simulink model "DCE_motor6_V2"  (R2025a)
settings: Solver=ode4  StartTime=0.0  StopTime=1  FixedStep=5e-5  RelTol=1e-3
undefined symbols (not defined in the file or in its folder): powergui
libraries: spsControlledVoltageSourceLib x24, spsControlledCurrentSourceLib x24, spsVoltageMeasurementLib x24, slpidlib x24, spspowerguiLib x2, simulink x1
(part 5 of 5)

== system DCE_motor6_V2/powergui1/EquivalentModel22/Sources ==
  Mux : Mux  Inputs=[1 1]
  u : Outport  VectorParamsAs1DForOutWhenUnconnected=off
  wires:
  Mux/1 -> u/1
  [T52_4806_4456650309996] -> Mux/1
  [T69_6431_8097857549454] -> Mux/2

== system DCE_motor6_V2/powergui1/EquivalentModel22/Yout ==
  v,i : Inport
  Demux : Demux  Outputs=1
  tag scope: T65_6117_7580539398846=global
  wires:
  v,i/1 -> Demux/1
  Demux/1 -> [T65_6117_7580539398846]

== system DCE_motor6_V2/powergui1/EquivalentModel23/Sources ==
  Mux : Mux  Inputs=[1 1]
  u : Outport  VectorParamsAs1DForOutWhenUnconnected=off
  wires:
  Mux/1 -> u/1
  [T52_4807_4456647609302] -> Mux/1
  [T68_6383_8137968106251] -> Mux/2

== system DCE_motor6_V2/powergui1/EquivalentModel23/Yout ==
  v,i : Inport
  Demux : Demux  Outputs=1
  tag scope: T64_6069_7569106032292=global
  wires:
  v,i/1 -> Demux/1
  Demux/1 -> [T64_6069_7569106032292]

== system DCE_motor6_V2/powergui1/EquivalentModel24/Sources ==
  Mux : Mux  Inputs=[1 1]
  u : Outport  VectorParamsAs1DForOutWhenUnconnected=off
  wires:
  Mux/1 -> u/1
  [T52_4808_4456787087070] -> Mux/1
  [T69_6432_8095244640554] -> Mux/2

== system DCE_motor6_V2/powergui1/EquivalentModel24/Yout ==
  v,i : Inport
  Demux : Demux  Outputs=1
  tag scope: T65_6118_7577934536865=global
  wires:
  v,i/1 -> Demux/1
  Demux/1 -> [T65_6118_7577934536865]

== system DCE_motor6_V2/powergui1/EquivalentModel3/Sources ==
  Mux : Mux  Inputs=[1 1]
  u : Outport  VectorParamsAs1DForOutWhenUnconnected=off
  wires:
  Mux/1 -> u/1
  [T52_4802_4466065559397] -> Mux/1
  [T68_6378_8149266987715] -> Mux/2

== system DCE_motor6_V2/powergui1/EquivalentModel3/Yout ==
  v,i : Inport
  Demux : Demux  Outputs=1
  tag scope: T64_6064_7580471701128=global
  wires:
  v,i/1 -> Demux/1
  Demux/1 -> [T64_6064_7580471701128]

== system DCE_motor6_V2/powergui1/EquivalentModel4/Sources ==
  Mux : Mux  Inputs=[1 1]
  u : Outport  VectorParamsAs1DForOutWhenUnconnected=off
  wires:
  Mux/1 -> u/1
  [T52_4803_4466210929170] -> Mux/1
  [T69_6427_8106398489851] -> Mux/2

== system DCE_motor6_V2/powergui1/EquivalentModel4/Yout ==
  v,i : Inport
  Demux : Demux  Outputs=1
  tag scope: T65_6113_7589152605399=global
  wires:
  v,i/1 -> Demux/1
  Demux/1 -> [T65_6113_7589152605399]

== system DCE_motor6_V2/powergui1/EquivalentModel5/Sources ==
  Mux : Mux  Inputs=[1 1]
  u : Outport  VectorParamsAs1DForOutWhenUnconnected=off
  wires:
  Mux/1 -> u/1
  [T52_4801_4464269315094] -> Mux/1
  [T68_6378_8149612899368] -> Mux/2

== system DCE_motor6_V2/powergui1/EquivalentModel5/Yout ==
  v,i : Inport
  Demux : Demux  Outputs=1
  tag scope: T64_6064_7580793483403=global
  wires:
  v,i/1 -> Demux/1
  Demux/1 -> [T64_6064_7580793483403]

== system DCE_motor6_V2/powergui1/EquivalentModel6/Sources ==
  Mux : Mux  Inputs=[1 1]
  u : Outport  VectorParamsAs1DForOutWhenUnconnected=off
  wires:
  Mux/1 -> u/1
  [T52_4802_4464129149544] -> Mux/1
  [T69_6427_8106740814706] -> Mux/2

== system DCE_motor6_V2/powergui1/EquivalentModel6/Yout ==
  v,i : Inport
  Demux : Demux  Outputs=1
  tag scope: T65_6113_7589471488212=global
  wires:
  v,i/1 -> Demux/1
  Demux/1 -> [T65_6113_7589471488212]

== system DCE_motor6_V2/powergui1/EquivalentModel7/Sources ==
  Mux : Mux  Inputs=[1 1]
  u : Outport  VectorParamsAs1DForOutWhenUnconnected=off
  wires:
  Mux/1 -> u/1
  [T52_4803_4464131162455] -> Mux/1
  [T68_6379_8146968359069] -> Mux/2

== system DCE_motor6_V2/powergui1/EquivalentModel7/Yout ==
  v,i : Inport
  Demux : Demux  Outputs=1
  tag scope: T64_6065_7578157286736=global
  wires:
  v,i/1 -> Demux/1
  Demux/1 -> [T64_6065_7578157286736]

== system DCE_motor6_V2/powergui1/EquivalentModel8/Sources ==
  Mux : Mux  Inputs=[1 1]
  u : Outport  VectorParamsAs1DForOutWhenUnconnected=off
  wires:
  Mux/1 -> u/1
  [T52_4804_4464275353827] -> Mux/1
  [T69_6428_8104129430716] -> Mux/2

== system DCE_motor6_V2/powergui1/EquivalentModel8/Yout ==
  v,i : Inport
  Demux : Demux  Outputs=1
  tag scope: T65_6114_7586868346154=global
  wires:
  v,i/1 -> Demux/1
  Demux/1 -> [T65_6114_7586868346154]

== system DCE_motor6_V2/powergui1/EquivalentModel9/Sources ==
  Mux : Mux  Inputs=[1 1]
  u : Outport  VectorParamsAs1DForOutWhenUnconnected=off
  wires:
  Mux/1 -> u/1
  [T52_4802_4462362678416] -> Mux/1
  [T68_6379_8147334089506] -> Mux/2

== system DCE_motor6_V2/powergui1/EquivalentModel9/Yout ==
  v,i : Inport
  Demux : Demux  Outputs=1
  tag scope: T64_6065_7578500152954=global
  wires:
  v,i/1 -> Demux/1
  Demux/1 -> [T64_6065_7578500152954]

== matlab function DCE_motor6_V2/joint6/MATLAB Function3 ==
  settings: updateMethod=DISCRETE
  data: iq input; TL_est output; wm input; theta_m input
function TL_est = fcn_Load_Observer(iq, wm, theta_m)
    % 步进电机实时负载转矩观测器 (基于 SVF 动态提取)
    % 控制周期: 5e-5 s

    persistent Ts p_pairs Psi_f B J Td;
    persistent a b alpha;
    persistent wf_p T_drive_f_p;

    if isempty(Ts)
        Ts = 5e-5;
        p_pairs = 50;
        
        % --- 【在此填入你的已知常量】 ---
        Psi_f = 0.0015;      % 已知磁链 (Wb)
        B = 1e-4;           % 已知粘滞摩擦系数 (N.m.s/rad)
        J = 1e-5;          % 已知转动惯量 (kg.m^2) (瞬态极重要！)
        Td = 0.003;          % 齿槽转矩幅值 (N.m) (填你模型里的实际值)
        
        % --- SVF 滤波器设计 ---
        % 截止频率设为 200Hz，足以滤除噪声，同时保留负载突变的动态响应
        f_c = 20;           
        alpha = 2 * pi * f_c;
        a = exp(-alpha * Ts);
        b = 1 - a;

        % 历史状态初始化
        wf_p = 0;
        T_drive_f_p = 0;
    end

    % 1. 计算总电磁生成转矩 Te
    T_main = p_pairs * Psi_f * iq;
    T_detent = -Td * sin(4 * p_pairs * theta_m);
    Te = T_main + T_detent;

    % 2. 计算纯驱动力矩 (扣除摩擦阻力)
    % T_drive = Te - B*w 
    T_drive = Te - B * wm;

    % 3. SVF 低通滤波 (平滑转速和驱动力矩)
    wf = a * wf_p + b * wm;
    T_drive_f = a * T_drive_f_p + b * T_drive;

    % 4. SVF 魔法：提取无噪声的角加速度 (dw/dt)
    dw_dt_est = alpha * (wm - wf_p);

    % 5. 计算实时负载转矩
    % TL = T_drive_filtered - J * (dw/dt)
    TL_est = T_drive_f - J * dw_dt_est;

    % 更新历史状态
    wf_p = wf;
    T_drive_f_p = T_drive_f;
end

== matlab function DCE_motor6_V2/joint6/MATLAB Function4 ==
  settings: updateMethod=DISCRETE  sampleTime=5e-5
  data: pos_ref_rad input; I_mag output; pos_real_rad input; vel_ref_rads input; vel_real_rads input; kp input; kv input; ki input; kd input
function I_mag = dce_controller(pos_ref_rad, pos_real_rad, vel_ref_rads, vel_real_rads, kp, kv, ki, kd)
    % 1. 单位转换
    rad2step = 51200 / (2 * pi); 
    pos_ref = pos_ref_rad * rad2step;
    pos_real = pos_real_rad * rad2step;
    vel_ref = vel_ref_rads * rad2step;
    
    % 【撤销滤波，恢复直接获取平滑的积分反馈速度】
    vel_real = vel_real_rads * rad2step; 
    
    % 3. 模拟 C++ 里的积分累加器
    persistent outputKi integralRound
    if isempty(outputKi)
        outputKi = 0;
        integralRound = 0;
    end
    
    pError = pos_ref - pos_real;
    pError = max(min(pError, 3200), -3200); 
    
    vError = (vel_ref - vel_real) / 128; 
    vError = max(min(vError, 4000), -4000); 
    
    outputKp = kp * pError;
    outputKd = kd * vError;
    
    integralRound = integralRound + (ki * pError + kv * vError);
    outputKi = outputKi + (integralRound / 128);
    integralRound = 0; 
    
    outputKi = max(min(outputKi, 1024000), -1024000); 
    
    output = (outputKp + outputKi + outputKd) / 1024; 
    output = max(min(output, 1000), -1000); 
    I_mag = output / 1000; 
end

== matlab function DCE_motor6_V2/joint6/Park1 ==
  data: Ia input; Id output; Ib input; Theta_elec input; Iq output
function [Id, Iq] = fcn(Ia, Ib, Theta_elec)
    Id =  Ia * cos(Theta_elec) + Ib * sin(Theta_elec);
    Iq = -Ia * sin(Theta_elec) + Ib * cos(Theta_elec);
end

== matlab function DCE_motor6_V2/joint6/Park2 ==
  data: Ia input; Id output; Ib input; Theta_elec input; Iq output
function [Id, Iq] = fcn(Ia, Ib, Theta_elec)
    Id =  Ia * cos(Theta_elec) + Ib * sin(Theta_elec);
    Iq = -Ia * sin(Theta_elec) + Ib * cos(Theta_elec);
end

== matlab function DCE_motor6_V2/joint6/RevPark1 ==
  data: Vq input; Vd input; Va_raw output; Theta_elec input; Vb_raw output
function [Va_raw, Vb_raw] = fcn(Vq, Vd, Theta_elec)
    Va_raw = Vd * cos(Theta_elec) - Vq * sin(Theta_elec);
    Vb_raw = Vd * sin(Theta_elec) + Vq * cos(Theta_elec);
end

== matlab function DCE_motor6_V2/joint2/MATLAB Function2 ==
  settings: updateMethod=DISCRETE  sampleTime=5e-5
  data: pos_ref_rad input; I_mag output; pos_real_rad input; vel_ref_rads input; vel_real_rads input; kp input; kv input; ki input; kd input
function I_mag = dce_controller(pos_ref_rad, pos_real_rad, vel_ref_rads, vel_real_rads, kp, kv, ki, kd)
    % 1. 单位转换
    rad2step = 51200 / (2 * pi); 
    pos_ref = pos_ref_rad * rad2step;
    pos_real = pos_real_rad * rad2step;
    vel_ref = vel_ref_rads * rad2step;
    
    % 【撤销滤波，恢复直接获取平滑的积分反馈速度】
    vel_real = vel_real_rads * rad2step; 
    
    % 3. 模拟 C++ 里的积分累加器
    persistent outputKi integralRound
    if isempty(outputKi)
        outputKi = 0;
        integralRound = 0;
    end
    
    pError = pos_ref - pos_real;
    pError = max(min(pError, 3200), -3200); 
    
    vError = (vel_ref - vel_real) / 128; 
    vError = max(min(vError, 4000), -4000); 
    
    outputKp = kp * pError;
    outputKd = kd * vError;
    
    integralRound = integralRound + (ki * pError + kv * vError);
    outputKi = outputKi + (integralRound / 128);
    integralRound = 0; 
    
    outputKi = max(min(outputKi, 1024000), -1024000); 
    
    output = (outputKp + outputKi + outputKd) / 1024; 
    output = max(min(output, 1000), -1000); 
    I_mag = output / 1000; 
end

== matlab function DCE_motor6_V2/joint6/RevPark2 ==
  data: Vq input; Vd input; Va_raw output; Theta_elec input; Vb_raw output
function [Va_raw, Vb_raw] = fcn(Vq, Vd, Theta_elec)
    Va_raw = Vd * cos(Theta_elec) - Vq * sin(Theta_elec);
    Vb_raw = Vd * sin(Theta_elec) + Vq * cos(Theta_elec);
end

== matlab function DCE_motor6_V2/joint3/MATLAB Function2 ==
  settings: updateMethod=DISCRETE  sampleTime=5e-5
  data: pos_ref_rad input; I_mag output; pos_real_rad input; vel_ref_rads input; vel_real_rads input; kp input; kv input; ki input; kd input
function I_mag = dce_controller(pos_ref_rad, pos_real_rad, vel_ref_rads, vel_real_rads, kp, kv, ki, kd)
    % 1. 单位转换
    rad2step = 51200 / (2 * pi); 
    pos_ref = pos_ref_rad * rad2step;
    pos_real = pos_real_rad * rad2step;
    vel_ref = vel_ref_rads * rad2step;
    
    % 【撤销滤波，恢复直接获取平滑的积分反馈速度】
    vel_real = vel_real_rads * rad2step; 
    
    % 3. 模拟 C++ 里的积分累加器
    persistent outputKi integralRound
    if isempty(outputKi)
        outputKi = 0;
        integralRound = 0;
    end
    
    pError = pos_ref - pos_real;
    pError = max(min(pError, 3200), -3200); 
    
    vError = (vel_ref - vel_real) / 128; 
    vError = max(min(vError, 4000), -4000); 
    
    outputKp = kp * pError;
    outputKd = kd * vError;
    
    integralRound = integralRound + (ki * pError + kv * vError);
    outputKi = outputKi + (integralRound / 128);
    integralRound = 0; 
    
    outputKi = max(min(outputKi, 1024000), -1024000); 
    
    output = (outputKp + outputKi + outputKd) / 1024; 
    output = max(min(output, 1000), -1000); 
    I_mag = output / 1000; 
end

== matlab function DCE_motor6_V2/joint3/MATLAB Function3 ==
  settings: updateMethod=DISCRETE
  data: iq input; TL_est output; wm input; theta_m input
function TL_est = fcn_Load_Observer(iq, wm, theta_m)
    % 步进电机实时负载转矩观测器 (基于 SVF 动态提取)
    % 控制周期: 5e-5 s

    persistent Ts p_pairs Psi_f B J Td;
    persistent a b alpha;
    persistent wf_p T_drive_f_p;

    if isempty(Ts)
        Ts = 5e-5;
        p_pairs = 50;
        
        % --- 【在此填入你的已知常量】 ---
        Psi_f = 0.0015;      % 已知磁链 (Wb)
        B = 1e-4;           % 已知粘滞摩擦系数 (N.m.s/rad)
        J = 1e-5;          % 已知转动惯量 (kg.m^2) (瞬态极重要！)
        Td = 0.003;          % 齿槽转矩幅值 (N.m) (填你模型里的实际值)
        
        % --- SVF 滤波器设计 ---
        % 截止频率设为 200Hz，足以滤除噪声，同时保留负载突变的动态响应
        f_c = 20;           
        alpha = 2 * pi * f_c;
        a = exp(-alpha * Ts);
        b = 1 - a;

        % 历史状态初始化
        wf_p = 0;
        T_drive_f_p = 0;
    end

    % 1. 计算总电磁生成转矩 Te
    T_main = p_pairs * Psi_f * iq;
    T_detent = -Td * sin(4 * p_pairs * theta_m);
    Te = T_main + T_detent;

    % 2. 计算纯驱动力矩 (扣除摩擦阻力)
    % T_drive = Te - B*w 
    T_drive = Te - B * wm;

    % 3. SVF 低通滤波 (平滑转速和驱动力矩)
    wf = a * wf_p + b * wm;
    T_drive_f = a * T_drive_f_p + b * T_drive;

    % 4. SVF 魔法：提取无噪声的角加速度 (dw/dt)
    dw_dt_est = alpha * (wm - wf_p);

    % 5. 计算实时负载转矩
    % TL = T_drive_filtered - J * (dw/dt)
    TL_est = T_drive_f - J * dw_dt_est;

    % 更新历史状态
    wf_p = wf;
    T_drive_f_p = T_drive_f;
end

== matlab function DCE_motor6_V2/joint3/MATLAB Function4 ==
  settings: updateMethod=DISCRETE  sampleTime=5e-5
  data: pos_ref_rad input; I_mag output; pos_real_rad input; vel_ref_rads input; vel_real_rads input; kp input; kv input; ki input; kd input
function I_mag = dce_controller(pos_ref_rad, pos_real_rad, vel_ref_rads, vel_real_rads, kp, kv, ki, kd)
    % 1. 单位转换
    rad2step = 51200 / (2 * pi); 
    pos_ref = pos_ref_rad * rad2step;
    pos_real = pos_real_rad * rad2step;
    vel_ref = vel_ref_rads * rad2step;
    
    % 【撤销滤波，恢复直接获取平滑的积分反馈速度】
    vel_real = vel_real_rads * rad2step; 
    
    % 3. 模拟 C++ 里的积分累加器
    persistent outputKi integralRound
    if isempty(outputKi)
        outputKi = 0;
        integralRound = 0;
    end
    
    pError = pos_ref - pos_real;
    pError = max(min(pError, 3200), -3200); 
    
    vError = (vel_ref - vel_real) / 128; 
    vError = max(min(vError, 4000), -4000); 
    
    outputKp = kp * pError;
    outputKd = kd * vError;
    
    integralRound = integralRound + (ki * pError + kv * vError);
    outputKi = outputKi + (integralRound / 128);
    integralRound = 0; 
    
    outputKi = max(min(outputKi, 1024000), -1024000); 
    
    output = (outputKp + outputKi + outputKd) / 1024; 
    output = max(min(output, 1000), -1000); 
    I_mag = output / 1000; 
end

== matlab function DCE_motor6_V2/joint3/Park1 ==
  data: Ia input; Id output; Ib input; Theta_elec input; Iq output
function [Id, Iq] = fcn(Ia, Ib, Theta_elec)
    Id =  Ia * cos(Theta_elec) + Ib * sin(Theta_elec);
    Iq = -Ia * sin(Theta_elec) + Ib * cos(Theta_elec);
end

== matlab function DCE_motor6_V2/MATLAB Function ==
  data: q input; pos_xyz output
function pos_xyz = forward_kinematics_sim(q)
    % 1. 机械臂物理参数 (直接内置，保证 Simulink 实时运行的独立性)
    p = [
        -0.019225  -0.000523   0.100684;
        -0.0155     0.035      0.0285;
         0.03665    0          0.146;
        -0.01855   -0.01       0.052;
         0.0168     0.127      0;
        -0.018506   0.077     -0.000106
    ];
    ax = [
         0  0 -1;
        -1  0  0;
        -1  0  0;
         0 -1  0;
        -1  0  0;
         0 -1  0
    ];

    % 2. 齐次变换矩阵连乘
    T_end = eye(4);
    for i = 1:6
        % 平移矩阵
        T_trans = eye(4); 
        T_trans(1:3,4) = p(i,:)';
        
        % 旋转轴
        u = ax(i,:); 
        u = u/norm(u);
        ux=u(1); uy=u(2); uz=u(3);
        
        % 当前关节角 (确保传入的是弧度 rad)
        th = q(i)*pi/180; 
        c = cos(th); s = sin(th); v = 1 - c;

        % 罗德里格斯旋转公式
        R = [ux^2*v+c,      ux*uy*v-uz*s,  ux*uz*v+uy*s;
             ux*uy*v+uz*s,  uy^2*v+c,      uy*uz*v-ux*s;
             ux*uz*v-uy*s,  uy*uz*v+ux*s,  uz^2*v+c];

        T_rot = eye(4); 
        T_rot(1:3,1:3) = R;
        
        % 累乘到末端
        T_end = T_end * (T_trans * T_rot);
    end

    % 3. 提取并输出末端笛卡尔坐标 [X; Y; Z]
    pos_xyz = T_end(1:3, 4);
end

== matlab function DCE_motor6_V2/joint3/Park2 ==
  data: Ia input; Id output; Ib input; Theta_elec input; Iq output
function [Id, Iq] = fcn(Ia, Ib, Theta_elec)
    Id =  Ia * cos(Theta_elec) + Ib * sin(Theta_elec);
    Iq = -Ia * sin(Theta_elec) + Ib * cos(Theta_elec);
end

== matlab function DCE_motor6_V2/joint1/MATLAB Function2 ==
  settings: updateMethod=DISCRETE  sampleTime=5e-5
  data: pos_ref_rad input; I_mag output; pos_real_rad input; vel_ref_rads input; vel_real_rads input; kp input; kv input; ki input; kd input
function I_mag = dce_controller(pos_ref_rad, pos_real_rad, vel_ref_rads, vel_real_rads, kp, kv, ki, kd)
    % 1. 单位转换
    rad2step = 51200 / (2 * pi); 
    pos_ref = pos_ref_rad * rad2step;
    pos_real = pos_real_rad * rad2step;
    vel_ref = vel_ref_rads * rad2step;
    
    % 【撤销滤波，恢复直接获取平滑的积分反馈速度】
    vel_real = vel_real_rads * rad2step; 
    
    % 3. 模拟 C++ 里的积分累加器
    persistent outputKi integralRound
    if isempty(outputKi)
        outputKi = 0;
        integralRound = 0;
    end
    
    pError = pos_ref - pos_real;
    pError = max(min(pError, 3200), -3200); 
    
    vError = (vel_ref - vel_real) / 128; 
    vError = max(min(vError, 4000), -4000); 
    
    outputKp = kp * pError;
    outputKd = kd * vError;
    
    integralRound = integralRound + (ki * pError + kv * vError);
    outputKi = outputKi + (integralRound / 128);
    integralRound = 0; 
    
    outputKi = max(min(outputKi, 1024000), -1024000); 
    
    output = (outputKp + outputKi + outputKd) / 1024; 
    output = max(min(output, 1000), -1000); 
    I_mag = output / 1000; 
end

== matlab function DCE_motor6_V2/joint1/MATLAB Function3 ==
  settings: updateMethod=DISCRETE
  data: iq input; TL_est output; wm input; theta_m input
function TL_est = fcn_Load_Observer(iq, wm, theta_m)
    % 步进电机实时负载转矩观测器 (基于 SVF 动态提取)
    % 控制周期: 5e-5 s

    persistent Ts p_pairs Psi_f B J Td;
    persistent a b alpha;
    persistent wf_p T_drive_f_p;

    if isempty(Ts)
        Ts = 5e-5;
        p_pairs = 50;
        
        % --- 【在此填入你的已知常量】 ---
        Psi_f = 0.0015;      % 已知磁链 (Wb)
        B = 1e-4;           % 已知粘滞摩擦系数 (N.m.s/rad)
        J = 1e-5;          % 已知转动惯量 (kg.m^2) (瞬态极重要！)
        Td = 0.003;          % 齿槽转矩幅值 (N.m) (填你模型里的实际值)
        
        % --- SVF 滤波器设计 ---
        % 截止频率设为 200Hz，足以滤除噪声，同时保留负载突变的动态响应
        f_c = 200;           
        alpha = 2 * pi * f_c;
        a = exp(-alpha * Ts);
        b = 1 - a;

        % 历史状态初始化
        wf_p = 0;
        T_drive_f_p = 0;
    end

    % 1. 计算总电磁生成转矩 Te
    T_main = p_pairs * Psi_f * iq;
    T_detent = -Td * sin(4 * p_pairs * theta_m);
    Te = T_main + T_detent;

    % 2. 计算纯驱动力矩 (扣除摩擦阻力)
    % T_drive = Te - B*w 
    T_drive = Te - B * wm;

    % 3. SVF 低通滤波 (平滑转速和驱动力矩)
    wf = a * wf_p + b * wm;
    T_drive_f = a * T_drive_f_p + b * T_drive;

    % 4. SVF 魔法：提取无噪声的角加速度 (dw/dt)
    dw_dt_est = alpha * (wm - wf_p);

    % 5. 计算实时负载转矩
    % TL = T_drive_filtered - J * (dw/dt)
    TL_est = T_drive_f - J * dw_dt_est;

    % 更新历史状态
    wf_p = wf;
    T_drive_f_p = T_drive_f;
end

== matlab function DCE_motor6_V2/joint1/MATLAB Function4 ==
  settings: updateMethod=DISCRETE  sampleTime=5e-5
  data: pos_ref_rad input; I_mag output; pos_real_rad input; vel_ref_rads input; vel_real_rads input; kp input; kv input; ki input; kd input
function I_mag = dce_controller(pos_ref_rad, pos_real_rad, vel_ref_rads, vel_real_rads, kp, kv, ki, kd)
    % 1. 单位转换
    rad2step = 51200 / (2 * pi); 
    pos_ref = pos_ref_rad * rad2step;
    pos_real = pos_real_rad * rad2step;
    vel_ref = vel_ref_rads * rad2step;
    
    % 【撤销滤波，恢复直接获取平滑的积分反馈速度】
    vel_real = vel_real_rads * rad2step; 
    
    % 3. 模拟 C++ 里的积分累加器
    persistent outputKi integralRound
    if isempty(outputKi)
        outputKi = 0;
        integralRound = 0;
    end
    
    pError = pos_ref - pos_real;
    pError = max(min(pError, 3200), -3200); 
    
    vError = (vel_ref - vel_real) / 128; 
    vError = max(min(vError, 4000), -4000); 
    
    outputKp = kp * pError;
    outputKd = kd * vError;
    
    integralRound = integralRound + (ki * pError + kv * vError);
    outputKi = outputKi + (integralRound / 128);
    integralRound = 0; 
    
    outputKi = max(min(outputKi, 1024000), -1024000); 
    
    output = (outputKp + outputKi + outputKd) / 1024; 
    output = max(min(output, 1000), -1000); 
    I_mag = output / 1000; 
end

== matlab function DCE_motor6_V2/joint1/Park1 ==
  data: Ia input; Id output; Ib input; Theta_elec input; Iq output
function [Id, Iq] = fcn(Ia, Ib, Theta_elec)
    Id =  Ia * cos(Theta_elec) + Ib * sin(Theta_elec);
    Iq = -Ia * sin(Theta_elec) + Ib * cos(Theta_elec);
end

== matlab function DCE_motor6_V2/joint1/Park2 ==
  data: Ia input; Id output; Ib input; Theta_elec input; Iq output
function [Id, Iq] = fcn(Ia, Ib, Theta_elec)
    Id =  Ia * cos(Theta_elec) + Ib * sin(Theta_elec);
    Iq = -Ia * sin(Theta_elec) + Ib * cos(Theta_elec);
end

== matlab function DCE_motor6_V2/joint2/MATLAB Function3 ==
  settings: updateMethod=DISCRETE
  data: iq input; TL_est output; wm input; theta_m input
function TL_est = fcn_Load_Observer(iq, wm, theta_m)
    % 步进电机实时负载转矩观测器 (基于 SVF 动态提取)
    % 控制周期: 5e-5 s

    persistent Ts p_pairs Psi_f B J Td;
    persistent a b alpha;
    persistent wf_p T_drive_f_p;

    if isempty(Ts)
        Ts = 5e-5;
        p_pairs = 50;
        
        % --- 【在此填入你的已知常量】 ---
        Psi_f = 0.0015;      % 已知磁链 (Wb)
        B = 1e-4;           % 已知粘滞摩擦系数 (N.m.s/rad)
        J = 1e-5;          % 已知转动惯量 (kg.m^2) (瞬态极重要！)
        Td = 0.003;          % 齿槽转矩幅值 (N.m) (填你模型里的实际值)
        
        % --- SVF 滤波器设计 ---
        % 截止频率设为 200Hz，足以滤除噪声，同时保留负载突变的动态响应
        f_c = 20;           
        alpha = 2 * pi * f_c;
        a = exp(-alpha * Ts);
        b = 1 - a;

        % 历史状态初始化
        wf_p = 0;
        T_drive_f_p = 0;
    end

    % 1. 计算总电磁生成转矩 Te
    T_main = p_pairs * Psi_f * iq;
    T_detent = -Td * sin(4 * p_pairs * theta_m);
    Te = T_main + T_detent;

    % 2. 计算纯驱动力矩 (扣除摩擦阻力)
    % T_drive = Te - B*w 
    T_drive = Te - B * wm;

    % 3. SVF 低通滤波 (平滑转速和驱动力矩)
    wf = a * wf_p + b * wm;
    T_drive_f = a * T_drive_f_p + b * T_drive;

    % 4. SVF 魔法：提取无噪声的角加速度 (dw/dt)
    dw_dt_est = alpha * (wm - wf_p);

    % 5. 计算实时负载转矩
    % TL = T_drive_filtered - J * (dw/dt)
    TL_est = T_drive_f - J * dw_dt_est;

    % 更新历史状态
    wf_p = wf;
    T_drive_f_p = T_drive_f;
end

== matlab function DCE_motor6_V2/joint1/RevPark1 ==
  data: Vq input; Vd input; Va_raw output; Theta_elec input; Vb_raw output
function [Va_raw, Vb_raw] = fcn(Vq, Vd, Theta_elec)
    Va_raw = Vd * cos(Theta_elec) - Vq * sin(Theta_elec);
    Vb_raw = Vd * sin(Theta_elec) + Vq * cos(Theta_elec);
end

== matlab function DCE_motor6_V2/joint1/RevPark2 ==
  data: Vq input; Vd input; Va_raw output; Theta_elec input; Vb_raw output
function [Va_raw, Vb_raw] = fcn(Vq, Vd, Theta_elec)
    Va_raw = Vd * cos(Theta_elec) - Vq * sin(Theta_elec);
    Vb_raw = Vd * sin(Theta_elec) + Vq * cos(Theta_elec);
end

== matlab function DCE_motor6_V2/joint3/RevPark1 ==
  data: Vq input; Vd input; Va_raw output; Theta_elec input; Vb_raw output
function [Va_raw, Vb_raw] = fcn(Vq, Vd, Theta_elec)
    Va_raw = Vd * cos(Theta_elec) - Vq * sin(Theta_elec);
    Vb_raw = Vd * sin(Theta_elec) + Vq * cos(Theta_elec);
end

== matlab function DCE_motor6_V2/joint3/RevPark2 ==
  data: Vq input; Vd input; Va_raw output; Theta_elec input; Vb_raw output
function [Va_raw, Vb_raw] = fcn(Vq, Vd, Theta_elec)
    Va_raw = Vd * cos(Theta_elec) - Vq * sin(Theta_elec);
    Vb_raw = Vd * sin(Theta_elec) + Vq * cos(Theta_elec);
end

== matlab function DCE_motor6_V2/joint4/MATLAB Function2 ==
  settings: updateMethod=DISCRETE  sampleTime=5e-5
  data: pos_ref_rad input; I_mag output; pos_real_rad input; vel_ref_rads input; vel_real_rads input; kp input; kv input; ki input; kd input
function I_mag = dce_controller(pos_ref_rad, pos_real_rad, vel_ref_rads, vel_real_rads, kp, kv, ki, kd)
    % 1. 单位转换
    rad2step = 51200 / (2 * pi); 
    pos_ref = pos_ref_rad * rad2step;
    pos_real = pos_real_rad * rad2step;
    vel_ref = vel_ref_rads * rad2step;
    
    % 【撤销滤波，恢复直接获取平滑的积分反馈速度】
    vel_real = vel_real_rads * rad2step; 
    
    % 3. 模拟 C++ 里的积分累加器
    persistent outputKi integralRound
    if isempty(outputKi)
        outputKi = 0;
        integralRound = 0;
    end
    
    pError = pos_ref - pos_real;
    pError = max(min(pError, 3200), -3200); 
    
    vError = (vel_ref - vel_real) / 128; 
    vError = max(min(vError, 4000), -4000); 
    
    outputKp = kp * pError;
    outputKd = kd * vError;
    
    integralRound = integralRound + (ki * pError + kv * vError);
    outputKi = outputKi + (integralRound / 128);
    integralRound = 0; 
    
    outputKi = max(min(outputKi, 1024000), -1024000); 
    
    output = (outputKp + outputKi + outputKd) / 1024; 
    output = max(min(output, 1000), -1000); 
    I_mag = output / 1000; 
end

== matlab function DCE_motor6_V2/joint4/MATLAB Function3 ==
  settings: updateMethod=DISCRETE
  data: iq input; TL_est output; wm input; theta_m input
function TL_est = fcn_Load_Observer(iq, wm, theta_m)
    % 步进电机实时负载转矩观测器 (基于 SVF 动态提取)
    % 控制周期: 5e-5 s

    persistent Ts p_pairs Psi_f B J Td;
    persistent a b alpha;
    persistent wf_p T_drive_f_p;

    if isempty(Ts)
        Ts = 5e-5;
        p_pairs = 50;
        
        % --- 【在此填入你的已知常量】 ---
        Psi_f = 0.0015;      % 已知磁链 (Wb)
        B = 1e-4;           % 已知粘滞摩擦系数 (N.m.s/rad)
        J = 1e-5;          % 已知转动惯量 (kg.m^2) (瞬态极重要！)
        Td = 0.003;          % 齿槽转矩幅值 (N.m) (填你模型里的实际值)
        
        % --- SVF 滤波器设计 ---
        % 截止频率设为 200Hz，足以滤除噪声，同时保留负载突变的动态响应
        f_c = 20;           
        alpha = 2 * pi * f_c;
        a = exp(-alpha * Ts);
        b = 1 - a;

        % 历史状态初始化
        wf_p = 0;
        T_drive_f_p = 0;
    end

    % 1. 计算总电磁生成转矩 Te
    T_main = p_pairs * Psi_f * iq;
    T_detent = -Td * sin(4 * p_pairs * theta_m);
    Te = T_main + T_detent;

    % 2. 计算纯驱动力矩 (扣除摩擦阻力)
    % T_drive = Te - B*w 
    T_drive = Te - B * wm;

    % 3. SVF 低通滤波 (平滑转速和驱动力矩)
    wf = a * wf_p + b * wm;
    T_drive_f = a * T_drive_f_p + b * T_drive;

    % 4. SVF 魔法：提取无噪声的角加速度 (dw/dt)
    dw_dt_est = alpha * (wm - wf_p);

    % 5. 计算实时负载转矩
    % TL = T_drive_filtered - J * (dw/dt)
    TL_est = T_drive_f - J * dw_dt_est;

    % 更新历史状态
    wf_p = wf;
    T_drive_f_p = T_drive_f;
end

== matlab function DCE_motor6_V2/joint4/MATLAB Function4 ==
  settings: updateMethod=DISCRETE  sampleTime=5e-5
  data: pos_ref_rad input; I_mag output; pos_real_rad input; vel_ref_rads input; vel_real_rads input; kp input; kv input; ki input; kd input
function I_mag = dce_controller(pos_ref_rad, pos_real_rad, vel_ref_rads, vel_real_rads, kp, kv, ki, kd)
    % 1. 单位转换
    rad2step = 51200 / (2 * pi); 
    pos_ref = pos_ref_rad * rad2step;
    pos_real = pos_real_rad * rad2step;
    vel_ref = vel_ref_rads * rad2step;
    
    % 【撤销滤波，恢复直接获取平滑的积分反馈速度】
    vel_real = vel_real_rads * rad2step; 
    
    % 3. 模拟 C++ 里的积分累加器
    persistent outputKi integralRound
    if isempty(outputKi)
        outputKi = 0;
        integralRound = 0;
    end
    
    pError = pos_ref - pos_real;
    pError = max(min(pError, 3200), -3200); 
    
    vError = (vel_ref - vel_real) / 128; 
    vError = max(min(vError, 4000), -4000); 
    
    outputKp = kp * pError;
    outputKd = kd * vError;
    
    integralRound = integralRound + (ki * pError + kv * vError);
    outputKi = outputKi + (integralRound / 128);
    integralRound = 0; 
    
    outputKi = max(min(outputKi, 1024000), -1024000); 
    
    output = (outputKp + outputKi + outputKd) / 1024; 
    output = max(min(output, 1000), -1000); 
    I_mag = output / 1000; 
end

== matlab function DCE_motor6_V2/joint4/Park1 ==
  data: Ia input; Id output; Ib input; Theta_elec input; Iq output
function [Id, Iq] = fcn(Ia, Ib, Theta_elec)
    Id =  Ia * cos(Theta_elec) + Ib * sin(Theta_elec);
    Iq = -Ia * sin(Theta_elec) + Ib * cos(Theta_elec);
end

== matlab function DCE_motor6_V2/joint4/Park2 ==
  data: Ia input; Id output; Ib input; Theta_elec input; Iq output
function [Id, Iq] = fcn(Ia, Ib, Theta_elec)
    Id =  Ia * cos(Theta_elec) + Ib * sin(Theta_elec);
    Iq = -Ia * sin(Theta_elec) + Ib * cos(Theta_elec);
end

== matlab function DCE_motor6_V2/joint2/MATLAB Function4 ==
  settings: updateMethod=DISCRETE  sampleTime=5e-5
  data: pos_ref_rad input; I_mag output; pos_real_rad input; vel_ref_rads input; vel_real_rads input; kp input; kv input; ki input; kd input
function I_mag = dce_controller(pos_ref_rad, pos_real_rad, vel_ref_rads, vel_real_rads, kp, kv, ki, kd)
    % 1. 单位转换
    rad2step = 51200 / (2 * pi); 
    pos_ref = pos_ref_rad * rad2step;
    pos_real = pos_real_rad * rad2step;
    vel_ref = vel_ref_rads * rad2step;
    
    % 【撤销滤波，恢复直接获取平滑的积分反馈速度】
    vel_real = vel_real_rads * rad2step; 
    
    % 3. 模拟 C++ 里的积分累加器
    persistent outputKi integralRound
    if isempty(outputKi)
        outputKi = 0;
        integralRound = 0;
    end
    
    pError = pos_ref - pos_real;
    pError = max(min(pError, 3200), -3200); 
    
    vError = (vel_ref - vel_real) / 128; 
    vError = max(min(vError, 4000), -4000); 
    
    outputKp = kp * pError;
    outputKd = kd * vError;
    
    integralRound = integralRound + (ki * pError + kv * vError);
    outputKi = outputKi + (integralRound / 128);
    integralRound = 0; 
    
    outputKi = max(min(outputKi, 1024000), -1024000); 
    
    output = (outputKp + outputKi + outputKd) / 1024; 
    output = max(min(output, 1000), -1000); 
    I_mag = output / 1000; 
end

== matlab function DCE_motor6_V2/joint4/RevPark1 ==
  data: Vq input; Vd input; Va_raw output; Theta_elec input; Vb_raw output
function [Va_raw, Vb_raw] = fcn(Vq, Vd, Theta_elec)
    Va_raw = Vd * cos(Theta_elec) - Vq * sin(Theta_elec);
    Vb_raw = Vd * sin(Theta_elec) + Vq * cos(Theta_elec);
end

== matlab function DCE_motor6_V2/joint4/RevPark2 ==
  data: Vq input; Vd input; Va_raw output; Theta_elec input; Vb_raw output
function [Va_raw, Vb_raw] = fcn(Vq, Vd, Theta_elec)
    Va_raw = Vd * cos(Theta_elec) - Vq * sin(Theta_elec);
    Vb_raw = Vd * sin(Theta_elec) + Vq * cos(Theta_elec);
end

== matlab function DCE_motor6_V2/joint5/MATLAB Function2 ==
  settings: updateMethod=DISCRETE  sampleTime=5e-5
  data: pos_ref_rad input; I_mag output; pos_real_rad input; vel_ref_rads input; vel_real_rads input; kp input; kv input; ki input; kd input
function I_mag = dce_controller(pos_ref_rad, pos_real_rad, vel_ref_rads, vel_real_rads, kp, kv, ki, kd)
    % 1. 单位转换
    rad2step = 51200 / (2 * pi); 
    pos_ref = pos_ref_rad * rad2step;
    pos_real = pos_real_rad * rad2step;
    vel_ref = vel_ref_rads * rad2step;
    
    % 【撤销滤波，恢复直接获取平滑的积分反馈速度】
    vel_real = vel_real_rads * rad2step; 
    
    % 3. 模拟 C++ 里的积分累加器
    persistent outputKi integralRound
    if isempty(outputKi)
        outputKi = 0;
        integralRound = 0;
    end
    
    pError = pos_ref - pos_real;
    pError = max(min(pError, 3200), -3200); 
    
    vError = (vel_ref - vel_real) / 128; 
    vError = max(min(vError, 4000), -4000); 
    
    outputKp = kp * pError;
    outputKd = kd * vError;
    
    integralRound = integralRound + (ki * pError + kv * vError);
    outputKi = outputKi + (integralRound / 128);
    integralRound = 0; 
    
    outputKi = max(min(outputKi, 1024000), -1024000); 
    
    output = (outputKp + outputKi + outputKd) / 1024; 
    output = max(min(output, 1000), -1000); 
    I_mag = output / 1000; 
end

== matlab function DCE_motor6_V2/joint5/MATLAB Function3 ==
  settings: updateMethod=DISCRETE
  data: iq input; TL_est output; wm input; theta_m input
function TL_est = fcn_Load_Observer(iq, wm, theta_m)
    % 步进电机实时负载转矩观测器 (基于 SVF 动态提取)
    % 控制周期: 5e-5 s

    persistent Ts p_pairs Psi_f B J Td;
    persistent a b alpha;
    persistent wf_p T_drive_f_p;

    if isempty(Ts)
        Ts = 5e-5;
        p_pairs = 50;
        
        % --- 【在此填入你的已知常量】 ---
        Psi_f = 0.0015;      % 已知磁链 (Wb)
        B = 1e-4;           % 已知粘滞摩擦系数 (N.m.s/rad)
        J = 1e-5;          % 已知转动惯量 (kg.m^2) (瞬态极重要！)
        Td = 0.003;          % 齿槽转矩幅值 (N.m) (填你模型里的实际值)
        
        % --- SVF 滤波器设计 ---
        % 截止频率设为 200Hz，足以滤除噪声，同时保留负载突变的动态响应
        f_c = 20;           
        alpha = 2 * pi * f_c;
        a = exp(-alpha * Ts);
        b = 1 - a;

        % 历史状态初始化
        wf_p = 0;
        T_drive_f_p = 0;
    end

    % 1. 计算总电磁生成转矩 Te
    T_main = p_pairs * Psi_f * iq;
    T_detent = -Td * sin(4 * p_pairs * theta_m);
    Te = T_main + T_detent;

    % 2. 计算纯驱动力矩 (扣除摩擦阻力)
    % T_drive = Te - B*w 
    T_drive = Te - B * wm;

    % 3. SVF 低通滤波 (平滑转速和驱动力矩)
    wf = a * wf_p + b * wm;
    T_drive_f = a * T_drive_f_p + b * T_drive;

    % 4. SVF 魔法：提取无噪声的角加速度 (dw/dt)
    dw_dt_est = alpha * (wm - wf_p);

    % 5. 计算实时负载转矩
    % TL = T_drive_filtered - J * (dw/dt)
    TL_est = T_drive_f - J * dw_dt_est;

    % 更新历史状态
    wf_p = wf;
    T_drive_f_p = T_drive_f;
end

== matlab function DCE_motor6_V2/joint5/MATLAB Function4 ==
  settings: updateMethod=DISCRETE  sampleTime=5e-5
  data: pos_ref_rad input; I_mag output; pos_real_rad input; vel_ref_rads input; vel_real_rads input; kp input; kv input; ki input; kd input
function I_mag = dce_controller(pos_ref_rad, pos_real_rad, vel_ref_rads, vel_real_rads, kp, kv, ki, kd)
    % 1. 单位转换
    rad2step = 51200 / (2 * pi); 
    pos_ref = pos_ref_rad * rad2step;
    pos_real = pos_real_rad * rad2step;
    vel_ref = vel_ref_rads * rad2step;
    
    % 【撤销滤波，恢复直接获取平滑的积分反馈速度】
    vel_real = vel_real_rads * rad2step; 
    
    % 3. 模拟 C++ 里的积分累加器
    persistent outputKi integralRound
    if isempty(outputKi)
        outputKi = 0;
        integralRound = 0;
    end
    
    pError = pos_ref - pos_real;
    pError = max(min(pError, 3200), -3200); 
    
    vError = (vel_ref - vel_real) / 128; 
    vError = max(min(vError, 4000), -4000); 
    
    outputKp = kp * pError;
    outputKd = kd * vError;
    
    integralRound = integralRound + (ki * pError + kv * vError);
    outputKi = outputKi + (integralRound / 128);
    integralRound = 0; 
    
    outputKi = max(min(outputKi, 1024000), -1024000); 
    
    output = (outputKp + outputKi + outputKd) / 1024; 
    output = max(min(output, 1000), -1000); 
    I_mag = output / 1000; 
end

== matlab function DCE_motor6_V2/joint5/Park1 ==
  data: Ia input; Id output; Ib input; Theta_elec input; Iq output
function [Id, Iq] = fcn(Ia, Ib, Theta_elec)
    Id =  Ia * cos(Theta_elec) + Ib * sin(Theta_elec);
    Iq = -Ia * sin(Theta_elec) + Ib * cos(Theta_elec);
end

== matlab function DCE_motor6_V2/joint5/Park2 ==
  data: Ia input; Id output; Ib input; Theta_elec input; Iq output
function [Id, Iq] = fcn(Ia, Ib, Theta_elec)
    Id =  Ia * cos(Theta_elec) + Ib * sin(Theta_elec);
    Iq = -Ia * sin(Theta_elec) + Ib * cos(Theta_elec);
end

== matlab function DCE_motor6_V2/joint5/RevPark1 ==
  data: Vq input; Vd input; Va_raw output; Theta_elec input; Vb_raw output
function [Va_raw, Vb_raw] = fcn(Vq, Vd, Theta_elec)
    Va_raw = Vd * cos(Theta_elec) - Vq * sin(Theta_elec);
    Vb_raw = Vd * sin(Theta_elec) + Vq * cos(Theta_elec);
end

== matlab function DCE_motor6_V2/joint5/RevPark2 ==
  data: Vq input; Vd input; Va_raw output; Theta_elec input; Vb_raw output
function [Va_raw, Vb_raw] = fcn(Vq, Vd, Theta_elec)
    Va_raw = Vd * cos(Theta_elec) - Vq * sin(Theta_elec);
    Vb_raw = Vd * sin(Theta_elec) + Vq * cos(Theta_elec);
end

== matlab function DCE_motor6_V2/MATLAB Function1 ==
  data: q input; pos_xyz output
function pos_xyz = forward_kinematics_sim(q)
    % 1. 机械臂物理参数 (直接内置，保证 Simulink 实时运行的独立性)
    p = [
        -0.019225  -0.000523   0.100684;
        -0.0155     0.035      0.0285;
         0.03665    0          0.146;
        -0.01855   -0.01       0.052;
         0.0168     0.127      0;
        -0.018506   0.077     -0.000106
    ];
    ax = [
         0  0 -1;
        -1  0  0;
        -1  0  0;
         0 -1  0;
        -1  0  0;
         0 -1  0
    ];

    % 2. 齐次变换矩阵连乘
    T_end = eye(4);
    for i = 1:6
        % 平移矩阵
        T_trans = eye(4); 
        T_trans(1:3,4) = p(i,:)';
        
        % 旋转轴
        u = ax(i,:); 
        u = u/norm(u);
        ux=u(1); uy=u(2); uz=u(3);
        
        % 当前关节角 (确保传入的是弧度 rad)
        th = q(i)*pi/180; 
        c = cos(th); s = sin(th); v = 1 - c;

        % 罗德里格斯旋转公式
        R = [ux^2*v+c,      ux*uy*v-uz*s,  ux*uz*v+uy*s;
             ux*uy*v+uz*s,  uy^2*v+c,      uy*uz*v-ux*s;
             ux*uz*v-uy*s,  uy*uz*v+ux*s,  uz^2*v+c];

        T_rot = eye(4); 
        T_rot(1:3,1:3) = R;
        
        % 累乘到末端
        T_end = T_end * (T_trans * T_rot);
    end

    % 3. 提取并输出末端笛卡尔坐标 [X; Y; Z]
    pos_xyz = T_end(1:3, 4);
end

== matlab function DCE_motor6_V2/MATLAB Function2 ==
  data: q input; pos_xyz output
function pos_xyz = forward_kinematics_sim(q)
    % 1. 机械臂物理参数 (直接内置，保证 Simulink 实时运行的独立性)
    p = [
        -0.019225  -0.000523   0.100684;
        -0.0155     0.035      0.0285;
         0.03665    0          0.146;
        -0.01855   -0.01       0.052;
         0.0168     0.127      0;
        -0.018506   0.077     -0.000106
    ];
    ax = [
         0  0 -1;
        -1  0  0;
        -1  0  0;
         0 -1  0;
        -1  0  0;
         0 -1  0
    ];

    % 2. 齐次变换矩阵连乘
    T_end = eye(4);
    for i = 1:6
        % 平移矩阵
        T_trans = eye(4); 
        T_trans(1:3,4) = p(i,:)';
        
        % 旋转轴
        u = ax(i,:); 
        u = u/norm(u);
        ux=u(1); uy=u(2); uz=u(3);
        
        % 当前关节角 (确保传入的是弧度 rad)
        th = q(i)*pi/180; 
        c = cos(th); s = sin(th); v = 1 - c;

        % 罗德里格斯旋转公式
        R = [ux^2*v+c,      ux*uy*v-uz*s,  ux*uz*v+uy*s;
             ux*uy*v+uz*s,  uy^2*v+c,      uy*uz*v-ux*s;
             ux*uz*v-uy*s,  uy*uz*v+ux*s,  uz^2*v+c];

        T_rot = eye(4); 
        T_rot(1:3,1:3) = R;
        
        % 累乘到末端
        T_end = T_end * (T_trans * T_rot);
    end

    % 3. 提取并输出末端笛卡尔坐标 [X; Y; Z]
    pos_xyz = T_end(1:3, 4);
end

== matlab function DCE_motor6_V2/joint2/Park1 ==
  data: Ia input; Id output; Ib input; Theta_elec input; Iq output
function [Id, Iq] = fcn(Ia, Ib, Theta_elec)
    Id =  Ia * cos(Theta_elec) + Ib * sin(Theta_elec);
    Iq = -Ia * sin(Theta_elec) + Ib * cos(Theta_elec);
end

== matlab function DCE_motor6_V2/joint2/Park2 ==
  data: Ia input; Id output; Ib input; Theta_elec input; Iq output
function [Id, Iq] = fcn(Ia, Ib, Theta_elec)
    Id =  Ia * cos(Theta_elec) + Ib * sin(Theta_elec);
    Iq = -Ia * sin(Theta_elec) + Ib * cos(Theta_elec);
end

== matlab function DCE_motor6_V2/joint2/RevPark1 ==
  data: Vq input; Vd input; Va_raw output; Theta_elec input; Vb_raw output
function [Va_raw, Vb_raw] = fcn(Vq, Vd, Theta_elec)
    Va_raw = Vd * cos(Theta_elec) - Vq * sin(Theta_elec);
    Vb_raw = Vd * sin(Theta_elec) + Vq * cos(Theta_elec);
end

== matlab function DCE_motor6_V2/joint2/RevPark2 ==
  data: Vq input; Vd input; Va_raw output; Theta_elec input; Vb_raw output
function [Va_raw, Vb_raw] = fcn(Vq, Vd, Theta_elec)
    Va_raw = Vd * cos(Theta_elec) - Vq * sin(Theta_elec);
    Vb_raw = Vd * sin(Theta_elec) + Vq * cos(Theta_elec);
end

== matlab function DCE_motor6_V2/joint6/MATLAB Function2 ==
  settings: updateMethod=DISCRETE  sampleTime=5e-5
  data: pos_ref_rad input; I_mag output; pos_real_rad input; vel_ref_rads input; vel_real_rads input; kp input; kv input; ki input; kd input
function I_mag = dce_controller(pos_ref_rad, pos_real_rad, vel_ref_rads, vel_real_rads, kp, kv, ki, kd)
    % 1. 单位转换
    rad2step = 51200 / (2 * pi); 
    pos_ref = pos_ref_rad * rad2step;
    pos_real = pos_real_rad * rad2step;
    vel_ref = vel_ref_rads * rad2step;
    
    % 【撤销滤波，恢复直接获取平滑的积分反馈速度】
    vel_real = vel_real_rads * rad2step; 
    
    % 3. 模拟 C++ 里的积分累加器
    persistent outputKi integralRound
    if isempty(outputKi)
        outputKi = 0;
        integralRound = 0;
    end
    
    pError = pos_ref - pos_real;
    pError = max(min(pError, 3200), -3200); 
    
    vError = (vel_ref - vel_real) / 128; 
    vError = max(min(vError, 4000), -4000); 
    
    outputKp = kp * pError;
    outputKd = kd * vError;
    
    integralRound = integralRound + (ki * pError + kv * vError);
    outputKi = outputKi + (integralRound / 128);
    integralRound = 0; 
    
    outputKi = max(min(outputKi, 1024000), -1024000); 
    
    output = (outputKp + outputKi + outputKd) / 1024; 
    output = max(min(output, 1000), -1000); 
    I_mag = output / 1000; 
end
